simulink library "INT_RmtAPP_VD"  (R2016b)
settings: Solver=VariableStepAuto  StartTime=0.0  StopTime=10.0  RelTol=1e-3
settings Model: Creator=bianxuyin  LastModifiedBy=bianxuyin

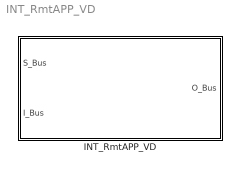
== system INT_RmtAPP_VD ==
  INT_RmtAPP_VD : Subsystem

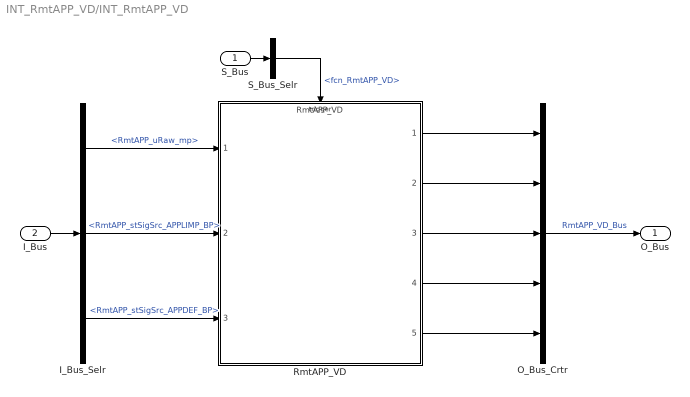
== system INT_RmtAPP_VD/INT_RmtAPP_VD ==
  S_Bus : Inport
  I_Bus : Inport  Port=2
  I_Bus_Selr : BusSelector  OutputSignals=RmtAPP_uRaw_mp,RmtAPP_stSigSrc_APPLIMP_BP,RmtAPP_stSigSrc_APPDEF_BP
  O_Bus_Crtr : BusCreator  Inputs=5
  RmtAPP_VD : ModelReference  ModelNameDialog=RmtAPP_VD  SimulationMode=Normal  ModelReferenceVersion=1.12  TriggerPortName=function  TriggerPortTriggerType=function-call  TriggerPortStatesWhenEnabling=held
  S_Bus_Selr : BusSelector  OutputSignals=fcn_RmtAPP_VD
  O_Bus : Outport
  wires:
  S_Bus_Selr/1 -> RmtAPP_VD/Trigger  "<fcn_RmtAPP_VD>"
  S_Bus/1 -> S_Bus_Selr/1
  I_Bus/1 -> I_Bus_Selr/1
  I_Bus_Selr/1 -> RmtAPP_VD/1  "<RmtAPP_uRaw_mp>"
  I_Bus_Selr/2 -> RmtAPP_VD/2  "<RmtAPP_stSigSrc_APPLIMP_BP>"
  I_Bus_Selr/3 -> RmtAPP_VD/3  "<RmtAPP_stSigSrc_APPDEF_BP>"
  O_Bus_Crtr/1 -> O_Bus/1  "RmtAPP_VD_Bus"
  RmtAPP_VD/1 -> O_Bus_Crtr/1
  RmtAPP_VD/2 -> O_Bus_Crtr/2
  RmtAPP_VD/3 -> O_Bus_Crtr/3
  RmtAPP_VD/4 -> O_Bus_Crtr/4
  RmtAPP_VD/5 -> O_Bus_Crtr/5
